simulink model "IK"  (R2020b)
settings: Solver=FixedStepAuto  StartTime=0.0  StopTime=inf  FixedStep=0.01  RelTol=1e-3  EnableMultiTasking=on
libraries: arduinolib x12
settings Model: SILPILModeSetting=veronly  ExtModeTrigDuration=2  Creator=Agc  LastModifiedBy=ali
settings OptimizationCC: EnhancedBackFolding=on  PassReuseOutputArgsAs=Individual arguments  ZeroExternalMemoryAtStartup=off  ZeroInternalMemoryAtStartup=off  MaxStackSize=64  OptimizeBlockOrder=speed  DifferentSizesBufferReuse=on  OptimizationCustomize=off  EfficientTunableParamExpr=on
settings DebuggingCC: ParameterTunabilityLossMsg=error
settings HardwareCC: ProdBitPerInt=16  ProdBitPerPointer=16  ProdBitPerSizeT=16  ProdBitPerPtrDiffT=16  ProdLargestAtomicFloat=None  ProdWordSize=8  ProdHWDeviceType=Atmel->AVR
settings SFSimCC: MATLABDynamicMemAlloc=off
settings RTWCC: Description=Embedded Coder  SystemTargetFile=ert.tlc  HardwareBoard=Arduino Mega 2560  TemplateMakefile=ert_default_tmf  GenerateReport=on  Toolchain=Arduino AVR  BuildConfiguration=Faster Runs  IncludeHyperlinkInReport=on  LaunchReport=on  GenerateTraceInfo=on  GenerateTraceReport=on  GenerateTraceReportSl=on  GenerateTraceReportSf=on  GenerateTraceReportEml=on
settings CodeAppCC: ForceParamTrailComments=on  IgnoreCustomStorageClasses=off  OperatorAnnotations=on  SimulinkDataObjDesc=on  SFDataObjDesc=on  InsertBlockDesc=on
settings ERTTargetCC: SupportContinuousTime=on  SupportVariableSizeSignals=on  ExtModeStaticAllocSize=2048

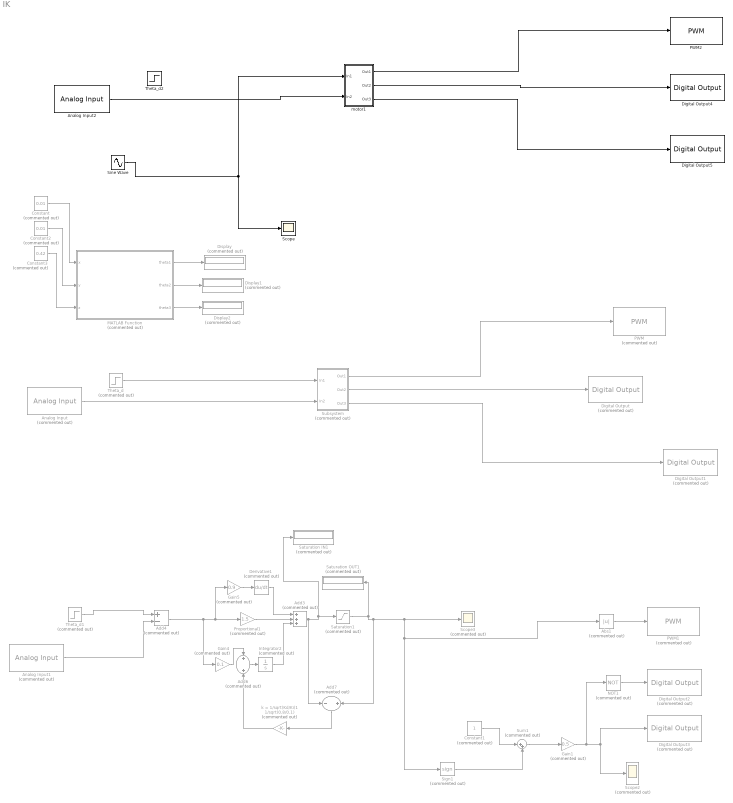
== system IK ==
  Abs1 : Abs  Commented=on
  Add3 : Sum  Commented=on  Inputs=+++
  Add4 : Sum  Commented=on  Inputs=+-
  Add6 : Sum  Commented=on
  Add7 : Sum  Commented=on  Inputs=-+
  Analog Input : arduinolib/Analog Input  Commented=on  pinNumber=1  ReadResultsOnly=off  ConversionTriggerSource=Software  ExternalTriggerType=uint32(0)  OutputDataType=uint16  EnableConversionCompleteNotify=off  EnableOuputStatus=off  SampleTime=-1  blockPlatform=arduino
  Analog Input1 : arduinolib/Analog Input  Commented=on  pinNumber=2  ReadResultsOnly=off  ConversionTriggerSource=Software  ExternalTriggerType=uint32(0)  OutputDataType=uint16  EnableConversionCompleteNotify=off  EnableOuputStatus=off  SampleTime=-1  blockPlatform=arduino
  Analog Input2 : arduinolib/Analog Input  pinNumber=0  ReadResultsOnly=off  ConversionTriggerSource=Software  ExternalTriggerType=uint32(0)  OutputDataType=uint16  EnableConversionCompleteNotify=off  EnableOuputStatus=off  SampleTime=-1  blockPlatform=arduino
  Constant : Constant  Commented=on  Value=0.01
  Constant1 : Constant  Commented=on
  Constant2 : Constant  Commented=on  Value=0.01
  Constant3 : Constant  Commented=on  Value=0.42
  Derivative1 : Derivative  Commented=on
  Digital Output : arduinolib/Digital Output  Commented=on  pinNumber=8  Direction=output  blockPlatform=arduino
  Digital Output1 : arduinolib/Digital Output  Commented=on  pinNumber=9  Direction=output  blockPlatform=arduino
  Digital Output2 : arduinolib/Digital Output  Commented=on  pinNumber=5  Direction=output  blockPlatform=arduino
  Digital Output3 : arduinolib/Digital Output  Commented=on  pinNumber=6  Direction=output  blockPlatform=arduino
  Digital Output4 : arduinolib/Digital Output  pinNumber=11  Direction=output  blockPlatform=arduino
  Digital Output5 : arduinolib/Digital Output  pinNumber=12  Direction=output  blockPlatform=arduino
  Display : Display  Commented=on
  Display1 : Display  Commented=on
  Display2 : Display  Commented=on
  Gain1 : Gain  Commented=on  Gain=0.5
  Gain4 : Gain  Commented=on  Gain=0.1
  Gain5 : Gain  Commented=on  Gain=0.9
  Integrator2 : Integrator  Commented=on
  MATLAB Function : MATLAB Function  Commented=on  TreatAsAtomicUnit=on
  NOT1 : Logic  Commented=on  Operator=NOT  IconShape=distinctive  AllPortsSameDT=off  OutDataTypeStr=boolean
  PWM : arduinolib/PWM  Commented=on  pinNumber=10  frequencyType=Default  desiredFrequency=490.2  achievableFrequency=490.2
  PWM1 : arduinolib/PWM  Commented=on  pinNumber=7  frequencyType=Default  desiredFrequency=490.2  achievableFrequency=490.2
  PWM2 : arduinolib/PWM  pinNumber=13  frequencyType=Default  desiredFrequency=490.2  achievableFrequency=490.2
  Proportional1 : Gain  Commented=on  Gain=1.5
  Saturation IN1 : Display  Commented=on
  Saturation OUT1 : Display  Commented=on
  Saturation1 : Saturate  Commented=on  UpperLimit=130  LowerLimit=-130
  Scope : Scope
  Scope2 : Scope  Commented=on
  Scope3 : Scope  Commented=on
  Sign1 : Signum  Commented=on
  Sine Wave : Sin  Amplitude=50  Bias=300  Frequency=3  SampleTime=0
  Subsystem : Subsystem  Commented=on
  Sum1 : Sum  Commented=on  Inputs=|++
  Theta_d : Step  Commented=on  After=180  SampleTime=0
  Theta_d1 : Step  Commented=on  After=95  SampleTime=0
  Theta_d2 : Step  SampleTime=0
  k = 1/sqrt(Kd/Ki)1 : Gain  Commented=on  Gain=1/sqrt(0.8/0.1)
  "motor1 " : Subsystem
  wires:
  Gain4/1 -> Add6/1
  Add7/1 -> k = 1/sqrt(Kd/Ki)1/1
  k = 1/sqrt(Kd/Ki)1/1 -> Add6/2
  Sum1/1 -> Gain1/1
  Abs1/1 -> PWM1/1
  Derivative1/1 -> Add3/1
  Proportional1/1 -> Add3/2
  Saturation1/1 -> Add7/2, Abs1/1, Sign1/1, Scope3/1, Saturation OUT1/1
  Add6/1 -> Integrator2/1
  Add3/1 -> Add7/1, Saturation IN1/1, Saturation1/1
  Gain5/1 -> Derivative1/1
  Analog Input1/1 -> Add4/2
  Add4/1 -> Gain5/1, Proportional1/1, Gain4/1
  NOT1/1 -> Digital Output2/1
  Sign1/1 -> Sum1/2
  Gain1/1 -> NOT1/1, Digital Output3/1, Scope2/1
  Theta_d1/1 -> Add4/1
  Constant1/1 -> Sum1/1
  Integrator2/1 -> Add3/3
  Analog Input2/1 -> "motor1 "/2(In2)
  "motor1 "/1(Out1) -> PWM2/1
  "motor1 "/2(Out2) -> Digital Output4/1
  "motor1 "/3(Out3) -> Digital Output5/1
  Theta_d/1 -> Subsystem/1(In1)
  Analog Input/1 -> Subsystem/2(In2)
  Subsystem/1(Out1) -> PWM/1
  Subsystem/2(Out2) -> Digital Output/1
  Subsystem/3(Out3) -> Digital Output1/1
  Sine Wave/1 -> Scope/1, "motor1 "/1(In1)
  Constant/1 -> MATLAB Function/1(x)
  Constant2/1 -> MATLAB Function/2(y)
  Constant3/1 -> MATLAB Function/3(z)
  MATLAB Function/1(theta1) -> Display/1
  MATLAB Function/2(theta2) -> Display1/1
  MATLAB Function/3(theta3) -> Display2/1

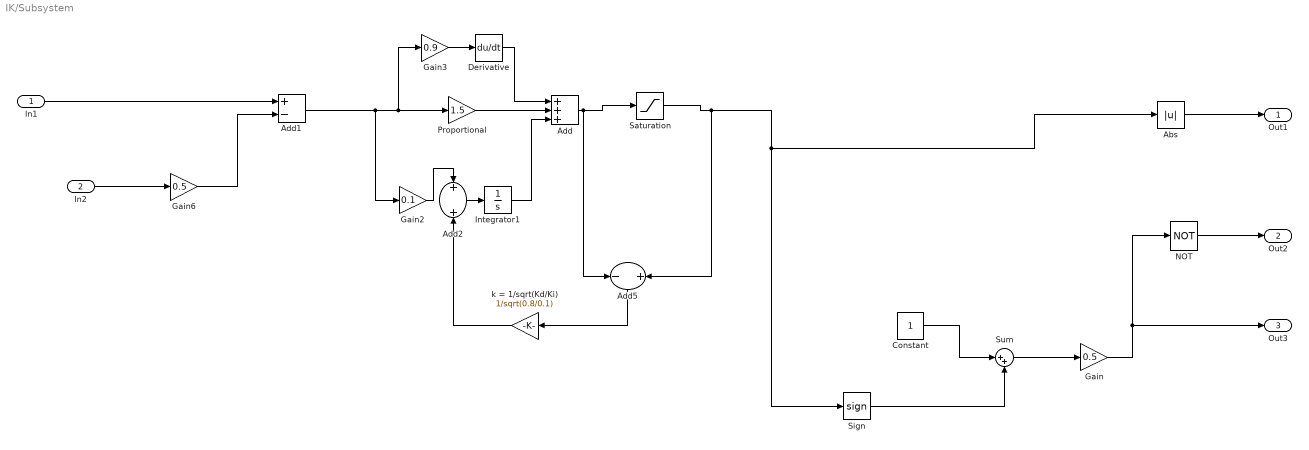
== system IK/Subsystem ==
  In1 : Inport
  In2 : Inport  Port=2
  Abs : Abs
  Add : Sum  Inputs=+++
  Add1 : Sum  Inputs=+-
  Add2 : Sum
  Add5 : Sum  Inputs=-+
  Constant : Constant
  Derivative : Derivative
  Gain : Gain  Gain=0.5
  Gain2 : Gain  Gain=0.1
  Gain3 : Gain  Gain=0.9
  Gain6 : Gain  Gain=0.5
  Integrator1 : Integrator
  NOT : Logic  Operator=NOT  IconShape=distinctive  AllPortsSameDT=off  OutDataTypeStr=boolean
  Proportional : Gain  Gain=1.5
  Saturation : Saturate  UpperLimit=130  LowerLimit=-130
  Sign : Signum
  Sum : Sum  Inputs=|++
  k = 1/sqrt(Kd/Ki) : Gain  Gain=1/sqrt(0.8/0.1)
  Out1 : Outport
  Out2 : Outport  Port=2
  Out3 : Outport  Port=3
  wires:
  In1/1 -> Add1/1
  Gain2/1 -> Add2/1
  Integrator1/1 -> Add/3
  Constant/1 -> Sum/1
  Add2/1 -> Integrator1/1
  Add1/1 -> Gain3/1, Proportional/1, Gain2/1
  Saturation/1 -> Add5/2, Abs/1, Sign/1
  Gain/1 -> Out3/1, NOT/1
  Gain6/1 -> Add1/2
  Add/1 -> Add5/1, Saturation/1
  In2/1 -> Gain6/1
  Sign/1 -> Sum/2
  Gain3/1 -> Derivative/1
  Proportional/1 -> Add/2
  Derivative/1 -> Add/1
  Sum/1 -> Gain/1
  k = 1/sqrt(Kd/Ki)/1 -> Add2/2
  Add5/1 -> k = 1/sqrt(Kd/Ki)/1
  NOT/1 -> Out2/1
  Abs/1 -> Out1/1

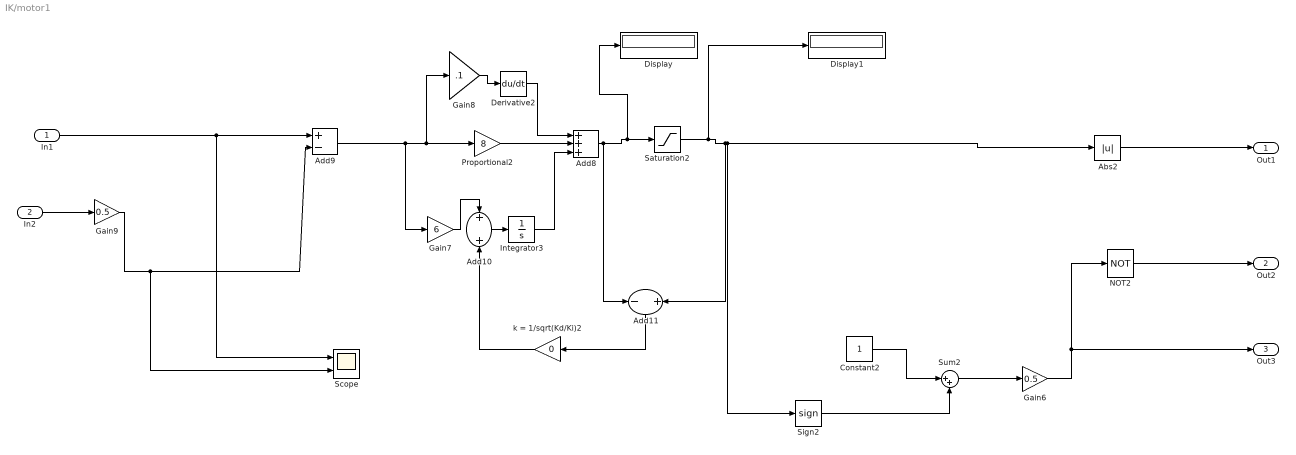
== system IK/motor1  ==
  In1 : Inport
  In2 : Inport  Port=2
  Abs2 : Abs
  Add10 : Sum
  Add11 : Sum  Inputs=-+
  Add8 : Sum  Inputs=+++
  Add9 : Sum  Inputs=+-
  Constant2 : Constant
  Derivative2 : Derivative
  Display : Display
  Display1 : Display
  Gain6 : Gain  Gain=0.5
  Gain7 : Gain  Gain=6
  Gain8 : Gain  Gain=.1
  Gain9 : Gain  Gain=0.5
  Integrator3 : Integrator
  NOT2 : Logic  Operator=NOT  IconShape=distinctive  AllPortsSameDT=off  OutDataTypeStr=boolean
  Proportional2 : Gain  Gain=8
  Saturation2 : Saturate  UpperLimit=130  LowerLimit=-130
  Scope : Scope  NumInputPorts=2
  Sign2 : Signum
  Sum2 : Sum  Inputs=|++
  k = 1/sqrt(Kd/Ki)2 : Gain  Gain=0
  Out1 : Outport
  Out2 : Outport  Port=2
  Out3 : Outport  Port=3
  wires:
  Proportional2/1 -> Add8/2
  Saturation2/1 -> Display1/1, Add11/2, Sign2/1, Abs2/1
  Derivative2/1 -> Add8/1
  Add9/1 -> Gain8/1, Proportional2/1, Gain7/1
  k = 1/sqrt(Kd/Ki)2/1 -> Add10/2
  Gain7/1 -> Add10/1
  Sum2/1 -> Gain6/1
  Add11/1 -> k = 1/sqrt(Kd/Ki)2/1
  Add8/1 -> Add11/1, Display/1, Saturation2/1
  Gain8/1 -> Derivative2/1
  Add10/1 -> Integrator3/1
  Abs2/1 -> Out1/1
  Sign2/1 -> Sum2/2
  Gain6/1 -> Out3/1, NOT2/1
  Integrator3/1 -> Add8/3
  Constant2/1 -> Sum2/1
  In2/1 -> Gain9/1
  NOT2/1 -> Out2/1
  In1/1 -> Scope/1, Add9/1
  Gain9/1 -> Add9/2, Scope/2

== matlab function IK/MATLAB Function ==
  data: x input; theta1 output; y input; z input; theta2 output; theta3 output
function [theta1, theta2, theta3] = inverse(x,y,z)
    d1 = 0.235;
    a2 = 0.13;
    a3 = 0.075;
    q1 = zeros(2,1);
    q3 = zeros(2,1);
    %theta1
    q1(1) = atan2(y,x);
    q1(2) = atan2(y,x) + pi;

    %theta3
    D = (x^2 + y^2 + (z - d1)^2 - (a2)^2 - (a3)^2)/(2 * a2 *a3);
    q3(1) = atan2(sqrt(1-D^2) , D);
    q3(2) = atan2(-sqrt(1-D^2) , D);

    %theta2
    q2 = atan2(z-d1, sqrt(x^2 + y^2)) - atan2(a3 * sin(q3(1)), a2 + a3 * cos(q3(1)));
    
    theta1 = q1(1);
    theta2 = q2;
    theta3 = q3(1);
